simulink model "punto4"  (Simulink 5.0)
settings: Solver=ode45  StartTime=0.0  StopTime=40  RelTol=1e-3
settings Model: LastModifiedBy=Juan

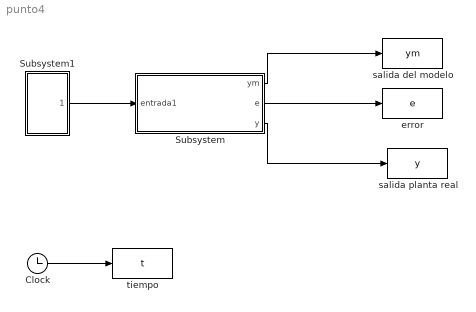
== system punto4 ==
  Clock : Clock
      settings: Decimation=10
  Subsystem : Subsystem  mask{kp=1, km=1, g1=0.1, titainicial=0}
      mask prompts: kp "ganancia de la planta real (kp)"; km "ganancia del modelo (km)"; g1 "gama1 (gama/b)"; titainicial "valor inicial de tita"
      mask Display: disp('Sistema')
  Subsystem1 : Subsystem  mask{w=1}
      mask prompts: w "Amplitud"
  error : ToWorkspace  VariableName=e  SampleTime=-1  SaveFormat=Array
  salida del modelo : ToWorkspace  VariableName=ym  SampleTime=-1  SaveFormat=Array
  salida planta real : ToWorkspace  VariableName=y  SampleTime=-1  SaveFormat=Array
  tiempo : ToWorkspace  VariableName=t  SampleTime=-1  SaveFormat=Array
  wires:
  Clock/1 -> tiempo/1
  Subsystem/1(ym) -> salida del modelo/1
  Subsystem1/1(Entrada) -> Subsystem/1(entrada1)
  Subsystem/2(e) -> error/1
  Subsystem/3(y) -> salida planta real/1

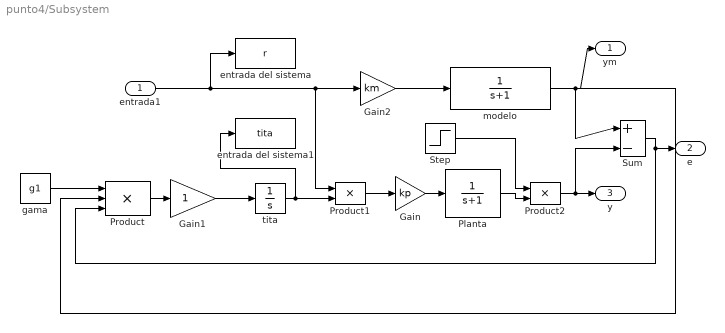
== system punto4/Subsystem ==
  entrada1 : Inport
  Gain : Gain  Gain=kp  SaturateOnIntegerOverflow=on
  Gain1 : Gain  SaturateOnIntegerOverflow=on
  Gain2 : Gain  Gain=km  SaturateOnIntegerOverflow=on
  Planta : TransferFcn  Numerator=1  Denominator=[1 1]
  Product : Product  Inputs=3  SaturateOnIntegerOverflow=on
  Product1 : Product  SaturateOnIntegerOverflow=on
  Product2 : Product  SaturateOnIntegerOverflow=on
  Step : Step  Time=20  Before=4  After=2  SampleTime=0
  Sum : Sum  Inputs=|+-  SaturateOnIntegerOverflow=on
  entrada del sistema : ToWorkspace  VariableName=r  SampleTime=-1  SaveFormat=Array
  entrada del sistema1 : ToWorkspace  VariableName=tita  SampleTime=-1  SaveFormat=Array
  gama : Constant  Value=g1
  modelo : TransferFcn  Numerator=1  Denominator=[1 1]
  tita : Integrator  InitialCondition=titainicial
  ym : Outport
  e : Outport  Port=2
  y : Outport  Port=3
  wires:
  Product/1 -> Gain1/1
  modelo/1 -> Sum/1, Product/2, ym/1
  Product1/1 -> Gain/1
  tita/1 -> Product1/2, entrada del sistema1/1
  Gain1/1 -> tita/1
  Sum/1 -> Product/3, e/1
  gama/1 -> Product/1
  Gain2/1 -> modelo/1
  Gain/1 -> Planta/1
  entrada1/1 -> entrada del sistema/1, Product1/1, Gain2/1
  Product2/1 -> y/1, Sum/2
  Planta/1 -> Product2/2
  Step/1 -> Product2/1

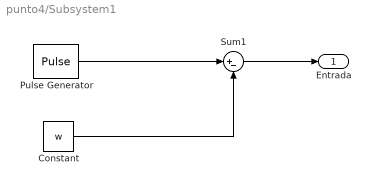
== system punto4/Subsystem1 ==
  Constant : Constant  Value=w
  Pulse Generator : DiscretePulseGenerator  PulseType=Time based  Amplitude=w*2  Period=20  PulseWidth=50
  Sum1 : Sum  Inputs=|+-  SaturateOnIntegerOverflow=on
  Entrada : Outport
  wires:
  Constant/1 -> Sum1/2
  Pulse Generator/1 -> Sum1/1
  Sum1/1 -> Entrada/1
